simulink model "ModelRikiRollCalib"  (R2015b)
settings: Solver=ode45  StartTime=0.0  StopTime=3  MaxStep=Ts  RelTol=1e-3
model workspace (MAT data in the model file):
  MCOS : class17 (value not decoded)
  MCOS : class17 (value not decoded)
  MCOS : class17 (value not decoded)
  MCOS : class17 (value not decoded)
  MCOS : class17 (value not decoded)
values from neighbouring files (symbols this model uses):
  AltKp = 0.03    [params.mat]
  AltRateBias = 0.65    [params.mat]
  AltRateKi = 0.01    [params.mat]
  AltRateKp = 0.05    [params.mat]
  AltRateMax = 6    [params.mat]
  FilterK = [0.01 0.01 0.01 0.01 0.01 0.01 0.01 0.01 0.01 0.01 0.01 0.01 ... (100 elements, 1x100)]    [params.mat]
  PosKp = 0.1    [params.mat]
  RollPitchKp = 10    [params.mat]
  RollPitchMax = 30    [params.mat]
  RollPitchRateKd = 5e-05    [params.mat]
  RollPitchRateKi = 0.002    [params.mat]
  RollPitchRateKp = 0.0007    [params.mat]
  RollPitchRateMax = 200    [params.mat]
  VelKi = 0.02    [params.mat]
  VelKp = 0.15    [params.mat]
  VelMax = 6    [params.mat]
  Waypts = [10 20 50 50 50 50 200 20 20 0 0 50 ... (27 elements, 9x3)]    [params.mat]
  YawKp = 3    [params.mat]
  YawRateKi = 0.000213867089849    [params.mat]
  YawRateKp = 0.00321759853461    [params.mat]
  YawRateMax = 180    [params.mat]
undefined symbols (not defined in the file or in its folder): DiscIntNeverNeededParam, Earth, Receive, RollPitchKd, Send, sigbuilder_block, WGS84
libraries: simulink x49, aerolibutil x8, simulink_extras x6, aerolibfltsims x5, aerolibanimutils x2, aerolibtransform2 x2, aerolibconvert2 x2, aerolib6dof2 x1, aerolibatmos2 x1
(part 2 of 3)

== system ModelRikiRollCalib/Ctrl/AutoCtrl/Roll Controller ==
  BUS : Inport
  RollRef : Inport  Port=2
  Bus Selector1 : BusSelector  OutputSignals=RPY,dRPY
  Discrete PID Controller : simulink/Continuous/PID Controller  Controller=PI  TimeDomain=Discrete-time  SampleTime=Ts  IntegratorMethod=Forward Euler  FilterMethod=Forward Euler  Form=Parallel  UseFilter=on  ControllerParametersSource=internal  P=RollPitchRateKp  I=RollPitchRateKi  D=0  N=50  InitialConditionSource=internal  InitialConditionForIntegrator=0  InitialConditionForFilter=0  ExternalReset=none  LimitOutput=on  UpperSaturationLimit=0.2  LowerSaturationLimit=-0.2  LinearizeAsGain=off  AntiWindupMode=clamping  Kb=1  TrackingMode=off  Kt=1  PParamMin=[]  PParamMax=[]  IParamMin=[]  IParamMax=[]  DParamMin=[]  DParamMax=[]  NParamMin=[]  NParamMax=[]  KbParamMin=[]  KbParamMax=[]  KtParamMin=[]  KtParamMax=[]  POutMin=[]  POutMax=[]  IOutMin=[]  IOutMax=[]  DOutMin=[]  DOutMax=[]  NOutMin=[]  NOutMax=[]  KbOutMin=[]  KbOutMax=[]  KtOutMin=[]  KtOutMax=[]  IntegratorOutMin=[]  IntegratorOutMax=[]  FilterOutMin=[]  FilterOutMax=[]  SumOutMin=[]  SumOutMax=[]  SumI1OutMin=[]  SumI1OutMax=[]  SumI2OutMin=[]  SumI2OutMax=[]  SumI3OutMin=[]  SumI3OutMax=[]  SumDOutMin=[]  SumDOutMax=[]  SaturationOutMin=[]  SaturationOutMax=[]  IntegratorContinuousStateAttributes=''  IntegratorStateMustResolveToSignalObject=off  IntegratorRTWStateStorageClass=Auto  FilterContinuousStateAttributes=''  FilterStateMustResolveToSignalObject=off  FilterRTWStateStorageClass=Auto  DifferentiatorICPrevScaledInput=0  DifferentiatorOutMin=[]  DifferentiatorOutMax=[]
  Discrete PID Controller1 : simulink/Continuous/PID Controller  Controller=P  TimeDomain=Discrete-time  SampleTime=Ts  IntegratorMethod=Forward Euler  FilterMethod=Forward Euler  Form=Parallel  UseFilter=on  ControllerParametersSource=internal  P=RollPitchKp  I=0.0227534008426031  D=0  N=50  InitialConditionSource=internal  InitialConditionForIntegrator=0  InitialConditionForFilter=0  ExternalReset=none  LimitOutput=on  UpperSaturationLimit=RollPitchRateMax  LowerSaturationLimit=-RollPitchRateMax  LinearizeAsGain=off  AntiWindupMode=clamping  Kb=1  TrackingMode=off  Kt=1  PParamMin=[]  PParamMax=[]  IParamMin=[]  IParamMax=[]  DParamMin=[]  DParamMax=[]  NParamMin=[]  NParamMax=[]  KbParamMin=[]  KbParamMax=[]  KtParamMin=[]  KtParamMax=[]  POutMin=[]  POutMax=[]  IOutMin=[]  IOutMax=[]  DOutMin=[]  DOutMax=[]  NOutMin=[]  NOutMax=[]  KbOutMin=[]  KbOutMax=[]  KtOutMin=[]  KtOutMax=[]  IntegratorOutMin=[]  IntegratorOutMax=[]  FilterOutMin=[]  FilterOutMax=[]  SumOutMin=[]  SumOutMax=[]  SumI1OutMin=[]  SumI1OutMax=[]  SumI2OutMin=[]  SumI2OutMax=[]  SumI3OutMin=[]  SumI3OutMax=[]  SumDOutMin=[]  SumDOutMax=[]  SaturationOutMin=[]  SaturationOutMax=[]  IntegratorContinuousStateAttributes=''  IntegratorStateMustResolveToSignalObject=off  IntegratorRTWStateStorageClass=Auto  FilterContinuousStateAttributes=''  FilterStateMustResolveToSignalObject=off  FilterRTWStateStorageClass=Auto  DifferentiatorICPrevScaledInput=0  DifferentiatorOutMin=[]  DifferentiatorOutMax=[]
  Scale roll2 : Gain  Gain=RollPitchMax
  Selector : Selector  InputPortWidth=3  IndexOptions=Index vector (dialog)  Indices=[1]  OutputSizes=1
  Selector3 : Selector  InputPortWidth=3  IndexOptions=Index vector (dialog)  Indices=[1]  OutputSizes=1
  Sum : Sum  Inputs=|+-
  Sum3 : Sum  Inputs=|+-
  RollPWM : Outport
  wires:
  Scale roll2/1 -> Sum3/1
  Sum3/1 -> Discrete PID Controller1/1
  Selector3/1 -> Sum3/2
  Discrete PID Controller1/1 -> Sum/1
  Bus Selector1/1 -> Selector3/1  "<RPY>"
  Sum/1 -> Discrete PID Controller/1
  RollRef/1 -> Scale roll2/1
  Discrete PID Controller/1 -> RollPWM/1
  Selector/1 -> Sum/2  "dRoll"
  Bus Selector1/2 -> Selector/1  "<dRPY>"
  BUS/1 -> Bus Selector1/1

== system ModelRikiRollCalib/Ctrl/AutoCtrl/Subsystem ==
  AltRef : Inport
  VertVel : Inport  Port=2
  Altitude : Inport  Port=3
  Bias1 : Bias  Bias=AltRateBias
  Discrete PID Controller1 : simulink/Continuous/PID Controller  Controller=PI  TimeDomain=Discrete-time  SampleTime=Ts  IntegratorMethod=Forward Euler  FilterMethod=Forward Euler  Form=Parallel  UseFilter=on  ControllerParametersSource=internal  P=AltRateKp  I=AltRateKi  D=0  N=50  InitialConditionSource=internal  InitialConditionForIntegrator=0  InitialConditionForFilter=0  ExternalReset=none  LimitOutput=on  UpperSaturationLimit=0.5  LowerSaturationLimit=-0.5  LinearizeAsGain=off  AntiWindupMode=clamping  Kb=1  TrackingMode=off  Kt=1  PParamMin=[]  PParamMax=[]  IParamMin=[]  IParamMax=[]  DParamMin=[]  DParamMax=[]  NParamMin=[]  NParamMax=[]  KbParamMin=[]  KbParamMax=[]  KtParamMin=[]  KtParamMax=[]  POutMin=[]  POutMax=[]  IOutMin=[]  IOutMax=[]  DOutMin=[]  DOutMax=[]  NOutMin=[]  NOutMax=[]  KbOutMin=[]  KbOutMax=[]  KtOutMin=[]  KtOutMax=[]  IntegratorOutMin=[]  IntegratorOutMax=[]  FilterOutMin=[]  FilterOutMax=[]  SumOutMin=[]  SumOutMax=[]  SumI1OutMin=[]  SumI1OutMax=[]  SumI2OutMin=[]  SumI2OutMax=[]  SumI3OutMin=[]  SumI3OutMax=[]  SumDOutMin=[]  SumDOutMax=[]  SaturationOutMin=[]  SaturationOutMax=[]  IntegratorContinuousStateAttributes=''  IntegratorStateMustResolveToSignalObject=off  IntegratorRTWStateStorageClass=Auto  FilterContinuousStateAttributes=''  FilterStateMustResolveToSignalObject=off  FilterRTWStateStorageClass=Auto  DifferentiatorICPrevScaledInput=0  DifferentiatorOutMin=[]  DifferentiatorOutMax=[]
  Discrete PID Controller2 : simulink/Continuous/PID Controller  Controller=P  TimeDomain=Discrete-time  SampleTime=Ts  IntegratorMethod=Forward Euler  FilterMethod=Forward Euler  Form=Parallel  UseFilter=on  ControllerParametersSource=internal  P=AltKp  I=AltRateKi  D=0  N=50  InitialConditionSource=internal  InitialConditionForIntegrator=0  InitialConditionForFilter=0  ExternalReset=none  LimitOutput=on  UpperSaturationLimit=0.5  LowerSaturationLimit=-0.5  LinearizeAsGain=off  AntiWindupMode=clamping  Kb=1  TrackingMode=off  Kt=1  PParamMin=[]  PParamMax=[]  IParamMin=[]  IParamMax=[]  DParamMin=[]  DParamMax=[]  NParamMin=[]  NParamMax=[]  KbParamMin=[]  KbParamMax=[]  KtParamMin=[]  KtParamMax=[]  POutMin=[]  POutMax=[]  IOutMin=[]  IOutMax=[]  DOutMin=[]  DOutMax=[]  NOutMin=[]  NOutMax=[]  KbOutMin=[]  KbOutMax=[]  KtOutMin=[]  KtOutMax=[]  IntegratorOutMin=[]  IntegratorOutMax=[]  FilterOutMin=[]  FilterOutMax=[]  SumOutMin=[]  SumOutMax=[]  SumI1OutMin=[]  SumI1OutMax=[]  SumI2OutMin=[]  SumI2OutMax=[]  SumI3OutMin=[]  SumI3OutMax=[]  SumDOutMin=[]  SumDOutMax=[]  SaturationOutMin=[]  SaturationOutMax=[]  IntegratorContinuousStateAttributes=''  IntegratorStateMustResolveToSignalObject=off  IntegratorRTWStateStorageClass=Auto  FilterContinuousStateAttributes=''  FilterStateMustResolveToSignalObject=off  FilterRTWStateStorageClass=Auto  DifferentiatorICPrevScaledInput=0  DifferentiatorOutMin=[]  DifferentiatorOutMax=[]
  Scale Vel : Gain  Gain=AltRateMax*2
  Sum1 : Sum  Inputs=|+-
  Sum3 : Sum  Inputs=|+-
  Out1 : Outport
  wires:
  Bias1/1 -> Out1/1
  Scale Vel/1 -> Sum3/1
  VertVel/1 -> Sum3/2
  Discrete PID Controller1/1 -> Bias1/1
  Sum3/1 -> Discrete PID Controller1/1
  AltRef/1 -> Sum1/1
  Altitude/1 -> Sum1/2
  Discrete PID Controller2/1 -> Scale Vel/1
  Sum1/1 -> Discrete PID Controller2/1

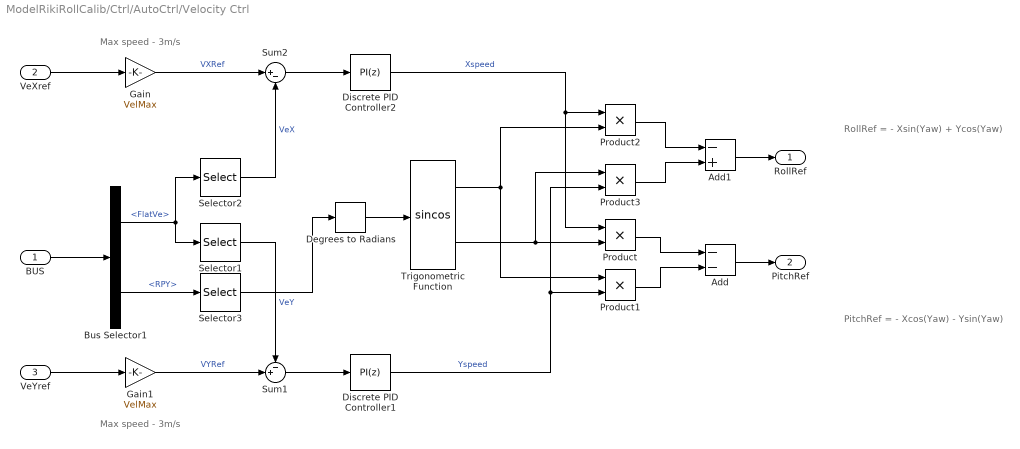
== system ModelRikiRollCalib/Ctrl/AutoCtrl/Velocity Ctrl ==
  note: Max speed - 3m/s
  note: PitchRef = - Xcos(Yaw) - Ysin(Yaw)
  note: RollRef = - Xsin(Yaw) + Ycos(Yaw)
  note: Max speed - 3m/s
  BUS : Inport
  VeXref : Inport  Port=2
  VeYref : Inport  Port=3
  Add : Sum  Inputs=--
  Add1 : Sum  Inputs=-+
  Bus Selector1 : BusSelector  OutputSignals=FlatVe,RPY
  Degrees to Radians : simulink_extras/Transformations/Degrees to Radians
  Discrete PID Controller1 : simulink/Continuous/PID Controller  Controller=PI  TimeDomain=Discrete-time  SampleTime=Ts  IntegratorMethod=Forward Euler  FilterMethod=Forward Euler  Form=Parallel  UseFilter=on  ControllerParametersSource=internal  P=VelKp  I=VelKi  D=0  N=50  InitialConditionSource=internal  InitialConditionForIntegrator=0  InitialConditionForFilter=0  ExternalReset=none  LimitOutput=on  UpperSaturationLimit=1  LowerSaturationLimit=-1  LinearizeAsGain=off  AntiWindupMode=clamping  Kb=1  TrackingMode=off  Kt=1  PParamMin=[]  PParamMax=[]  IParamMin=[]  IParamMax=[]  DParamMin=[]  DParamMax=[]  NParamMin=[]  NParamMax=[]  KbParamMin=[]  KbParamMax=[]  KtParamMin=[]  KtParamMax=[]  POutMin=[]  POutMax=[]  IOutMin=[]  IOutMax=[]  DOutMin=[]  DOutMax=[]  NOutMin=[]  NOutMax=[]  KbOutMin=[]  KbOutMax=[]  KtOutMin=[]  KtOutMax=[]  IntegratorOutMin=[]  IntegratorOutMax=[]  FilterOutMin=[]  FilterOutMax=[]  SumOutMin=[]  SumOutMax=[]  SumI1OutMin=[]  SumI1OutMax=[]  SumI2OutMin=[]  SumI2OutMax=[]  SumI3OutMin=[]  SumI3OutMax=[]  SumDOutMin=[]  SumDOutMax=[]  SaturationOutMin=[]  SaturationOutMax=[]  IntegratorContinuousStateAttributes=''  IntegratorStateMustResolveToSignalObject=off  IntegratorRTWStateStorageClass=Auto  FilterContinuousStateAttributes=''  FilterStateMustResolveToSignalObject=off  FilterRTWStateStorageClass=Auto  DifferentiatorICPrevScaledInput=0  DifferentiatorOutMin=[]  DifferentiatorOutMax=[]
  Discrete PID Controller2 : simulink/Continuous/PID Controller  Controller=PI  TimeDomain=Discrete-time  SampleTime=Ts  IntegratorMethod=Forward Euler  FilterMethod=Forward Euler  Form=Parallel  UseFilter=on  ControllerParametersSource=internal  P=VelKp  I=VelKi  D=0  N=50  InitialConditionSource=internal  InitialConditionForIntegrator=0  InitialConditionForFilter=0  ExternalReset=none  LimitOutput=on  UpperSaturationLimit=1  LowerSaturationLimit=-1  LinearizeAsGain=off  AntiWindupMode=clamping  Kb=1  TrackingMode=off  Kt=1  PParamMin=[]  PParamMax=[]  IParamMin=[]  IParamMax=[]  DParamMin=[]  DParamMax=[]  NParamMin=[]  NParamMax=[]  KbParamMin=[]  KbParamMax=[]  KtParamMin=[]  KtParamMax=[]  POutMin=[]  POutMax=[]  IOutMin=[]  IOutMax=[]  DOutMin=[]  DOutMax=[]  NOutMin=[]  NOutMax=[]  KbOutMin=[]  KbOutMax=[]  KtOutMin=[]  KtOutMax=[]  IntegratorOutMin=[]  IntegratorOutMax=[]  FilterOutMin=[]  FilterOutMax=[]  SumOutMin=[]  SumOutMax=[]  SumI1OutMin=[]  SumI1OutMax=[]  SumI2OutMin=[]  SumI2OutMax=[]  SumI3OutMin=[]  SumI3OutMax=[]  SumDOutMin=[]  SumDOutMax=[]  SaturationOutMin=[]  SaturationOutMax=[]  IntegratorContinuousStateAttributes=''  IntegratorStateMustResolveToSignalObject=off  IntegratorRTWStateStorageClass=Auto  FilterContinuousStateAttributes=''  FilterStateMustResolveToSignalObject=off  FilterRTWStateStorageClass=Auto  DifferentiatorICPrevScaledInput=0  DifferentiatorOutMin=[]  DifferentiatorOutMax=[]
  Gain : Gain  Gain=VelMax
  Gain1 : Gain  Gain=VelMax
  Product{,1..3} (4 alike) : Product  RndMeth=Zero
  Selector1 : Selector  InputPortWidth=3  IndexOptions=Index vector (dialog)  Indices=[2]  OutputSizes=1
  Selector2 : Selector  InputPortWidth=3  IndexOptions=Index vector (dialog)  Indices=[1]  OutputSizes=1
  Selector3 : Selector  InputPortWidth=3  IndexOptions=Index vector (dialog)  Indices=[3]  OutputSizes=1
  Sum1 : Sum  Inputs=-+|
  Sum2 : Sum  Inputs=|+-
  Trigonometric Function : Trigonometry  Operator=sincos
  RollRef : Outport
  PitchRef : Outport  Port=2
  wires:
  VeXref/1 -> Gain/1
  Selector2/1 -> Sum2/2  "VeX"
  Sum2/1 -> Discrete PID Controller2/1
  Bus Selector1/1 -> Selector1/1, Selector2/1  "<FlatVe>"
  BUS/1 -> Bus Selector1/1
  VeYref/1 -> Gain1/1
  Selector1/1 -> Sum1/1  "VeY"
  Sum1/1 -> Discrete PID Controller1/1
  Discrete PID Controller2/1 -> Product/1, Product2/1  "Xspeed"
  Discrete PID Controller1/1 -> Product1/2, Product3/2  "Yspeed"
  Trigonometric Function/2 -> Product/2, Product3/1
  Trigonometric Function/1 -> Product1/1, Product2/2
  Product1/1 -> Add/2
  Product/1 -> Add/1
  Product2/1 -> Add1/1
  Product3/1 -> Add1/2
  Add1/1 -> RollRef/1
  Add/1 -> PitchRef/1
  Bus Selector1/2 -> Selector3/1  "<RPY>"
  Selector3/1 -> Degrees to Radians/1
  Gain/1 -> Sum2/1  "VXRef"
  Gain1/1 -> Sum1/2  "VYRef"
  Degrees to Radians/1 -> Trigonometric Function/1

== system ModelRikiRollCalib/Ctrl/AutoCtrl/Yaw Controller ==
  BUS : Inport
  YawRef : Inport  Port=2
  Bus Selector3 : BusSelector  OutputSignals=RPY,dRPY
  Correct Yaw1 : MATLAB Function  TreatAsAtomicUnit=on
  Discrete PID Controller : simulink/Continuous/PID Controller  Controller=PI  TimeDomain=Discrete-time  SampleTime=Ts  IntegratorMethod=Forward Euler  FilterMethod=Forward Euler  Form=Parallel  UseFilter=on  ControllerParametersSource=internal  P=YawRateKp  I=YawRateKi  D=0  N=10  InitialConditionSource=internal  InitialConditionForIntegrator=0  InitialConditionForFilter=0  ExternalReset=none  LimitOutput=on  UpperSaturationLimit=0.2  LowerSaturationLimit=-0.2  LinearizeAsGain=off  AntiWindupMode=clamping  Kb=1  TrackingMode=off  Kt=1  PParamMin=[]  PParamMax=[]  IParamMin=[]  IParamMax=[]  DParamMin=[]  DParamMax=[]  NParamMin=[]  NParamMax=[]  KbParamMin=[]  KbParamMax=[]  KtParamMin=[]  KtParamMax=[]  POutMin=[]  POutMax=[]  IOutMin=[]  IOutMax=[]  DOutMin=[]  DOutMax=[]  NOutMin=[]  NOutMax=[]  KbOutMin=[]  KbOutMax=[]  KtOutMin=[]  KtOutMax=[]  IntegratorOutMin=[]  IntegratorOutMax=[]  FilterOutMin=[]  FilterOutMax=[]  SumOutMin=[]  SumOutMax=[]  SumI1OutMin=[]  SumI1OutMax=[]  SumI2OutMin=[]  SumI2OutMax=[]  SumI3OutMin=[]  SumI3OutMax=[]  SumDOutMin=[]  SumDOutMax=[]  SaturationOutMin=[]  SaturationOutMax=[]  IntegratorContinuousStateAttributes=''  IntegratorStateMustResolveToSignalObject=off  IntegratorRTWStateStorageClass=Auto  FilterContinuousStateAttributes=''  FilterStateMustResolveToSignalObject=off  FilterRTWStateStorageClass=Auto  DifferentiatorICPrevScaledInput=0  DifferentiatorOutMin=[]  DifferentiatorOutMax=[]
  Discrete PID Controller3 : simulink/Continuous/PID Controller  Controller=P  TimeDomain=Discrete-time  SampleTime=Ts  IntegratorMethod=Forward Euler  FilterMethod=Forward Euler  Form=Parallel  UseFilter=on  ControllerParametersSource=internal  P=YawKp  I=0  D=0  N=10  InitialConditionSource=internal  InitialConditionForIntegrator=0  InitialConditionForFilter=0  ExternalReset=none  LimitOutput=on  UpperSaturationLimit=YawRateMax  LowerSaturationLimit=-YawRateMax  LinearizeAsGain=off  AntiWindupMode=clamping  Kb=1  TrackingMode=off  Kt=1  PParamMin=[]  PParamMax=[]  IParamMin=[]  IParamMax=[]  DParamMin=[]  DParamMax=[]  NParamMin=[]  NParamMax=[]  KbParamMin=[]  KbParamMax=[]  KtParamMin=[]  KtParamMax=[]  POutMin=[]  POutMax=[]  IOutMin=[]  IOutMax=[]  DOutMin=[]  DOutMax=[]  NOutMin=[]  NOutMax=[]  KbOutMin=[]  KbOutMax=[]  KtOutMin=[]  KtOutMax=[]  IntegratorOutMin=[]  IntegratorOutMax=[]  FilterOutMin=[]  FilterOutMax=[]  SumOutMin=[]  SumOutMax=[]  SumI1OutMin=[]  SumI1OutMax=[]  SumI2OutMin=[]  SumI2OutMax=[]  SumI3OutMin=[]  SumI3OutMax=[]  SumDOutMin=[]  SumDOutMax=[]  SaturationOutMin=[]  SaturationOutMax=[]  IntegratorContinuousStateAttributes=''  IntegratorStateMustResolveToSignalObject=off  IntegratorRTWStateStorageClass=Auto  FilterContinuousStateAttributes=''  FilterStateMustResolveToSignalObject=off  FilterRTWStateStorageClass=Auto  DifferentiatorICPrevScaledInput=0  DifferentiatorOutMin=[]  DifferentiatorOutMax=[]
  Discrete-Time Integrator : DiscreteIntegrator  SampleTime=Ts  ICPrevOutput=DiscIntNeverNeededParam  ICPrevScaledInput=DiscIntNeverNeededParam
  Scale roll2 : Gain  Gain=90
  Selector : Selector  InputPortWidth=3  IndexOptions=Index vector (dialog)  Indices=[3]  OutputSizes=1
  Selector2 : Selector  InputPortWidth=3  IndexOptions=Index vector (dialog)  Indices=[3]  OutputSizes=1
  Sum : Sum  Inputs=|+-
  Sum3 : Sum  Inputs=|+-
  YawPWM : Outport
  wires:
  Scale roll2/1 -> Discrete-Time Integrator/1
  Selector2/1 -> Sum3/2
  YawRef/1 -> Scale roll2/1
  Bus Selector3/1 -> Selector2/1  "<RPY>"
  BUS/1 -> Bus Selector3/1
  Bus Selector3/2 -> Selector/1  "<dRPY>"
  Correct Yaw1/1(y) -> Discrete PID Controller3/1
  Discrete PID Controller3/1 -> Sum/1
  Sum3/1 -> Correct Yaw1/1(u)
  Selector/1 -> Sum/2  "dYaw"
  Sum/1 -> Discrete PID Controller/1
  Discrete PID Controller/1 -> YawPWM/1
  Discrete-Time Integrator/1 -> Sum3/1

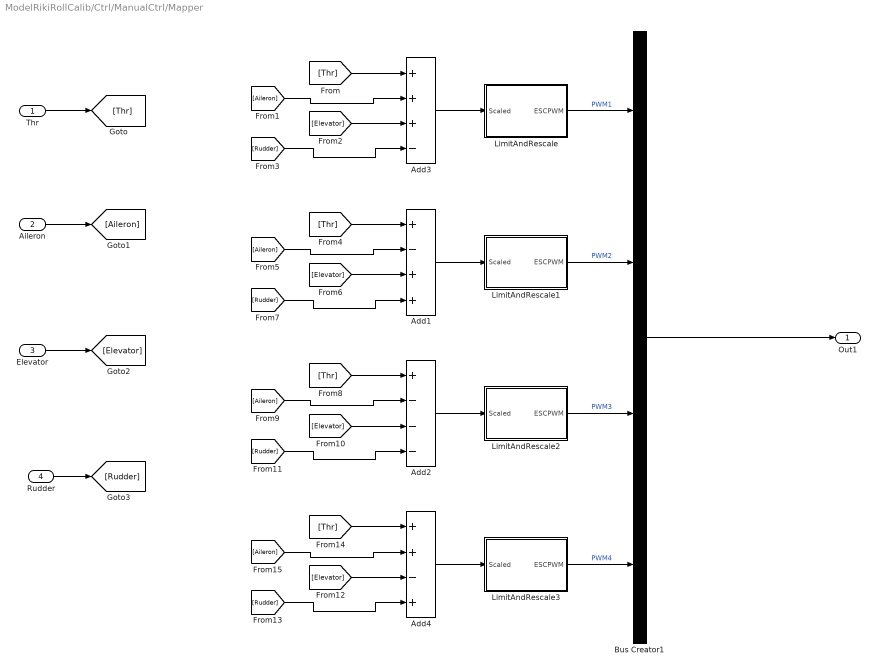
== system ModelRikiRollCalib/Ctrl/ManualCtrl/Mapper ==
  Thr : Inport
  Aileron : Inport  Port=2
  Elevator : Inport  Port=3
  Rudder : Inport  Port=4
  Add1 : Sum  Inputs=+-++
  Add2 : Sum  Inputs=+---
  Add3 : Sum  Inputs=+++-
  Add4 : Sum  Inputs=++-+
  Bus Creator1 : BusCreator  Inputs=4
  LimitAndRescale : Subsystem
  LimitAndRescale1 : Subsystem
  LimitAndRescale2 : Subsystem
  LimitAndRescale3 : Subsystem
  Out1 : Outport
  wires:
  LimitAndRescale3/1(ESCPWM) -> Bus Creator1/4  "PWM4"
  Add4/1 -> LimitAndRescale3/1(Scaled)
  LimitAndRescale2/1(ESCPWM) -> Bus Creator1/3  "PWM3"
  Add2/1 -> LimitAndRescale2/1(Scaled)
  Bus Creator1/1 -> Out1/1
  LimitAndRescale/1(ESCPWM) -> Bus Creator1/1  "PWM1"
  Add3/1 -> LimitAndRescale/1(Scaled)
  LimitAndRescale1/1(ESCPWM) -> Bus Creator1/2  "PWM2"
  Thr/1 -> [Thr]
  Aileron/1 -> [Aileron]
  Elevator/1 -> [Elevator]
  Rudder/1 -> [Rudder]
  [Thr] -> Add3/1
  [Aileron] -> Add3/2
  [Elevator] -> Add3/3
  [Rudder] -> Add3/4
  Add1/1 -> LimitAndRescale1/1(Scaled)
  [Thr] -> Add1/1
  [Aileron] -> Add1/2
  [Elevator] -> Add1/3
  [Rudder] -> Add1/4
  [Thr] -> Add2/1
  [Aileron] -> Add2/2
  [Elevator] -> Add2/3
  [Rudder] -> Add2/4
  [Thr] -> Add4/1
  [Aileron] -> Add4/2
  [Elevator] -> Add4/3
  [Rudder] -> Add4/4

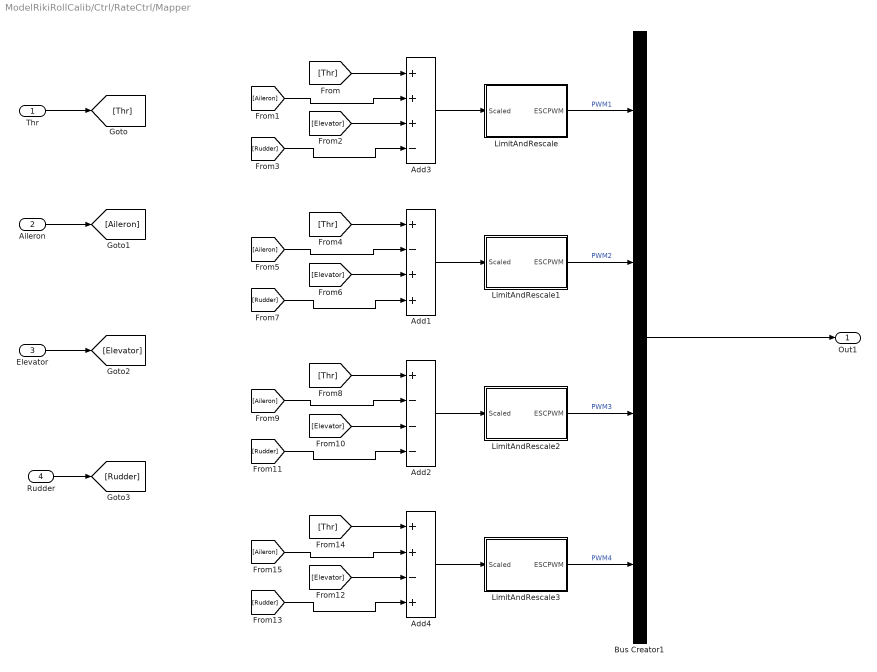
== system ModelRikiRollCalib/Ctrl/RateCtrl/Mapper ==
  Thr : Inport
  Aileron : Inport  Port=2
  Elevator : Inport  Port=3
  Rudder : Inport  Port=4
  Add1 : Sum  Inputs=+-++
  Add2 : Sum  Inputs=+---
  Add3 : Sum  Inputs=+++-
  Add4 : Sum  Inputs=++-+
  Bus Creator1 : BusCreator  Inputs=4
  LimitAndRescale : Subsystem
  LimitAndRescale1 : Subsystem
  LimitAndRescale2 : Subsystem
  LimitAndRescale3 : Subsystem
  Out1 : Outport
  wires:
  LimitAndRescale3/1(ESCPWM) -> Bus Creator1/4  "PWM4"
  Add4/1 -> LimitAndRescale3/1(Scaled)
  LimitAndRescale2/1(ESCPWM) -> Bus Creator1/3  "PWM3"
  Add2/1 -> LimitAndRescale2/1(Scaled)
  Bus Creator1/1 -> Out1/1
  LimitAndRescale/1(ESCPWM) -> Bus Creator1/1  "PWM1"
  Add3/1 -> LimitAndRescale/1(Scaled)
  LimitAndRescale1/1(ESCPWM) -> Bus Creator1/2  "PWM2"
  Thr/1 -> [Thr]
  Aileron/1 -> [Aileron]
  Elevator/1 -> [Elevator]
  Rudder/1 -> [Rudder]
  [Thr] -> Add3/1
  [Aileron] -> Add3/2
  [Elevator] -> Add3/3
  [Rudder] -> Add3/4
  Add1/1 -> LimitAndRescale1/1(Scaled)
  [Thr] -> Add1/1
  [Aileron] -> Add1/2
  [Elevator] -> Add1/3
  [Rudder] -> Add1/4
  [Thr] -> Add2/1
  [Aileron] -> Add2/2
  [Elevator] -> Add2/3
  [Rudder] -> Add2/4
  [Thr] -> Add4/1
  [Aileron] -> Add4/2
  [Elevator] -> Add4/3
  [Rudder] -> Add4/4

== system ModelRikiRollCalib/Ctrl/RateCtrl/Pitch Controller ==
  BUS : Inport
  PitchRef : Inport  Port=2
  Bus Selector1 : BusSelector  OutputSignals=dRPY
  Discrete PID Controller : simulink/Continuous/PID Controller  Controller=PI  TimeDomain=Discrete-time  SampleTime=Ts  IntegratorMethod=Forward Euler  FilterMethod=Forward Euler  Form=Parallel  UseFilter=on  ControllerParametersSource=internal  P=RollPitchRateKp  I=RollPitchRateKi  D=0  N=50  InitialConditionSource=internal  InitialConditionForIntegrator=0  InitialConditionForFilter=0  ExternalReset=none  LimitOutput=on  UpperSaturationLimit=0.2  LowerSaturationLimit=-0.2  LinearizeAsGain=off  AntiWindupMode=clamping  Kb=1  TrackingMode=off  Kt=1  PParamMin=[]  PParamMax=[]  IParamMin=[]  IParamMax=[]  DParamMin=[]  DParamMax=[]  NParamMin=[]  NParamMax=[]  KbParamMin=[]  KbParamMax=[]  KtParamMin=[]  KtParamMax=[]  POutMin=[]  POutMax=[]  IOutMin=[]  IOutMax=[]  DOutMin=[]  DOutMax=[]  NOutMin=[]  NOutMax=[]  KbOutMin=[]  KbOutMax=[]  KtOutMin=[]  KtOutMax=[]  IntegratorOutMin=[]  IntegratorOutMax=[]  FilterOutMin=[]  FilterOutMax=[]  SumOutMin=[]  SumOutMax=[]  SumI1OutMin=[]  SumI1OutMax=[]  SumI2OutMin=[]  SumI2OutMax=[]  SumI3OutMin=[]  SumI3OutMax=[]  SumDOutMin=[]  SumDOutMax=[]  SaturationOutMin=[]  SaturationOutMax=[]  IntegratorContinuousStateAttributes=''  IntegratorStateMustResolveToSignalObject=off  IntegratorRTWStateStorageClass=Auto  FilterContinuousStateAttributes=''  FilterStateMustResolveToSignalObject=off  FilterRTWStateStorageClass=Auto  DifferentiatorICPrevScaledInput=0  DifferentiatorOutMin=[]  DifferentiatorOutMax=[]
  Scale roll2 : Gain  Gain=RollPitchRateMax
  Selector : Selector  InputPortWidth=3  IndexOptions=Index vector (dialog)  Indices=[2]  OutputSizes=1
  Sum : Sum  Inputs=|+-
  PitchPWM : Outport
  wires:
  Scale roll2/1 -> Sum/1
  Sum/1 -> Discrete PID Controller/1
  PitchRef/1 -> Scale roll2/1
  Discrete PID Controller/1 -> PitchPWM/1
  Selector/1 -> Sum/2  "dPitch"
  Bus Selector1/1 -> Selector/1  "<dRPY>"
  BUS/1 -> Bus Selector1/1

== system ModelRikiRollCalib/Ctrl/RateCtrl/Roll Controller ==
  BUS : Inport
  RollRef : Inport  Port=2
  Bus Selector1 : BusSelector  OutputSignals=dRPY
  Discrete PID Controller : simulink/Continuous/PID Controller  Controller=PD  TimeDomain=Discrete-time  SampleTime=Ts  IntegratorMethod=Forward Euler  FilterMethod=Forward Euler  Form=Parallel  UseFilter=on  ControllerParametersSource=internal  P=RollPitchRateKp  I=RollPitchRateKi  D=RollPitchRateKd  N=50  InitialConditionSource=internal  InitialConditionForIntegrator=0  InitialConditionForFilter=0  ExternalReset=none  LimitOutput=on  UpperSaturationLimit=0.2  LowerSaturationLimit=-0.2  LinearizeAsGain=off  AntiWindupMode=clamping  Kb=1  TrackingMode=off  Kt=1  PParamMin=[]  PParamMax=[]  IParamMin=[]  IParamMax=[]  DParamMin=[]  DParamMax=[]  NParamMin=[]  NParamMax=[]  KbParamMin=[]  KbParamMax=[]  KtParamMin=[]  KtParamMax=[]  POutMin=[]  POutMax=[]  IOutMin=[]  IOutMax=[]  DOutMin=[]  DOutMax=[]  NOutMin=[]  NOutMax=[]  KbOutMin=[]  KbOutMax=[]  KtOutMin=[]  KtOutMax=[]  IntegratorOutMin=[]  IntegratorOutMax=[]  FilterOutMin=[]  FilterOutMax=[]  SumOutMin=[]  SumOutMax=[]  SumI1OutMin=[]  SumI1OutMax=[]  SumI2OutMin=[]  SumI2OutMax=[]  SumI3OutMin=[]  SumI3OutMax=[]  SumDOutMin=[]  SumDOutMax=[]  SaturationOutMin=[]  SaturationOutMax=[]  IntegratorContinuousStateAttributes=''  IntegratorStateMustResolveToSignalObject=off  IntegratorRTWStateStorageClass=Auto  FilterContinuousStateAttributes=''  FilterStateMustResolveToSignalObject=off  FilterRTWStateStorageClass=Auto  DifferentiatorICPrevScaledInput=0  DifferentiatorOutMin=[]  DifferentiatorOutMax=[]
  Scale roll2 : Gain  Gain=RollPitchRateMax
  Selector : Selector  InputPortWidth=3  IndexOptions=Index vector (dialog)  Indices=[1]  OutputSizes=1
  Sum : Sum  Inputs=|+-
  RollPWM : Outport
  wires:
  BUS/1 -> Bus Selector1/1
  Bus Selector1/1 -> Selector/1  "<dRPY>"
  Selector/1 -> Sum/2  "dRoll"
  Discrete PID Controller/1 -> RollPWM/1  "RateRollY"
  RollRef/1 -> Scale roll2/1
  Sum/1 -> Discrete PID Controller/1
  Scale roll2/1 -> Sum/1  "RateRollRef"

== system ModelRikiRollCalib/Ctrl/RateCtrl/Yaw Controller ==
  BUS : Inport
  YawRef : Inport  Port=2
  Bus Selector1 : BusSelector  OutputSignals=dRPY
  Discrete PID Controller : simulink/Continuous/PID Controller  Controller=PI  TimeDomain=Discrete-time  SampleTime=Ts  IntegratorMethod=Forward Euler  FilterMethod=Forward Euler  Form=Parallel  UseFilter=on  ControllerParametersSource=internal  P=YawRateKp  I=YawRateKi  D=0  N=10  InitialConditionSource=internal  InitialConditionForIntegrator=0  InitialConditionForFilter=0  ExternalReset=none  LimitOutput=on  UpperSaturationLimit=0.2  LowerSaturationLimit=-0.2  LinearizeAsGain=off  AntiWindupMode=clamping  Kb=1  TrackingMode=off  Kt=1  PParamMin=[]  PParamMax=[]  IParamMin=[]  IParamMax=[]  DParamMin=[]  DParamMax=[]  NParamMin=[]  NParamMax=[]  KbParamMin=[]  KbParamMax=[]  KtParamMin=[]  KtParamMax=[]  POutMin=[]  POutMax=[]  IOutMin=[]  IOutMax=[]  DOutMin=[]  DOutMax=[]  NOutMin=[]  NOutMax=[]  KbOutMin=[]  KbOutMax=[]  KtOutMin=[]  KtOutMax=[]  IntegratorOutMin=[]  IntegratorOutMax=[]  FilterOutMin=[]  FilterOutMax=[]  SumOutMin=[]  SumOutMax=[]  SumI1OutMin=[]  SumI1OutMax=[]  SumI2OutMin=[]  SumI2OutMax=[]  SumI3OutMin=[]  SumI3OutMax=[]  SumDOutMin=[]  SumDOutMax=[]  SaturationOutMin=[]  SaturationOutMax=[]  IntegratorContinuousStateAttributes=''  IntegratorStateMustResolveToSignalObject=off  IntegratorRTWStateStorageClass=Auto  FilterContinuousStateAttributes=''  FilterStateMustResolveToSignalObject=off  FilterRTWStateStorageClass=Auto  DifferentiatorICPrevScaledInput=0  DifferentiatorOutMin=[]  DifferentiatorOutMax=[]
  Scale roll2 : Gain  Gain=YawRateMax
  Selector : Selector  InputPortWidth=3  IndexOptions=Index vector (dialog)  Indices=[3]  OutputSizes=1
  Sum : Sum  Inputs=|+-
  YawPWM : Outport
  wires:
  Scale roll2/1 -> Sum/1
  Sum/1 -> Discrete PID Controller/1
  YawRef/1 -> Scale roll2/1
  Discrete PID Controller/1 -> YawPWM/1
  Selector/1 -> Sum/2  "dYaw"
  Bus Selector1/1 -> Selector/1  "<dRPY>"
  BUS/1 -> Bus Selector1/1

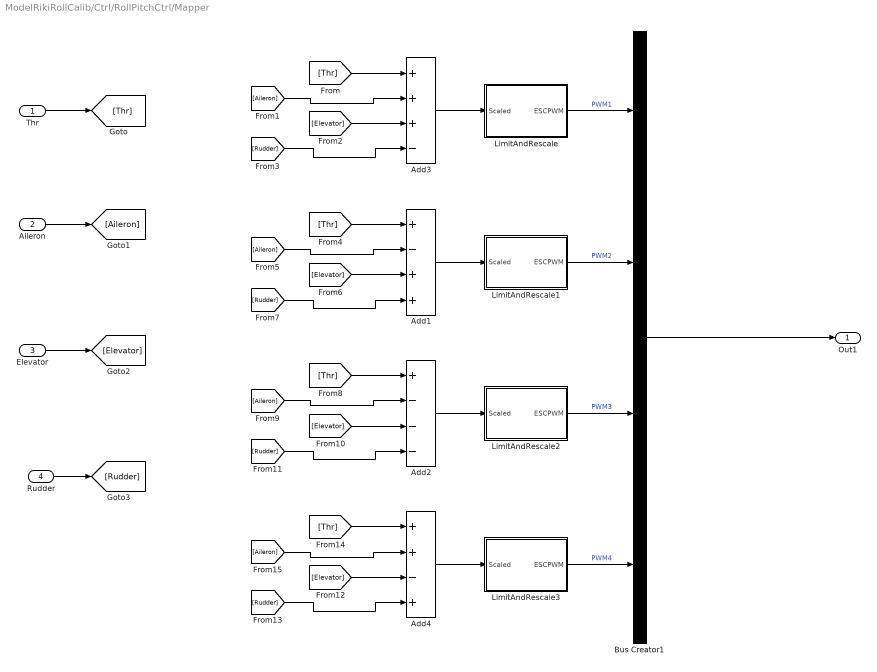
== system ModelRikiRollCalib/Ctrl/RollPitchCtrl/Mapper ==
  Thr : Inport
  Aileron : Inport  Port=2
  Elevator : Inport  Port=3
  Rudder : Inport  Port=4
  Add1 : Sum  Inputs=+-++
  Add2 : Sum  Inputs=+---
  Add3 : Sum  Inputs=+++-
  Add4 : Sum  Inputs=++-+
  Bus Creator1 : BusCreator  Inputs=4
  LimitAndRescale : Subsystem
  LimitAndRescale1 : Subsystem
  LimitAndRescale2 : Subsystem
  LimitAndRescale3 : Subsystem
  Out1 : Outport
  wires:
  LimitAndRescale3/1(ESCPWM) -> Bus Creator1/4  "PWM4"
  Add4/1 -> LimitAndRescale3/1(Scaled)
  LimitAndRescale2/1(ESCPWM) -> Bus Creator1/3  "PWM3"
  Add2/1 -> LimitAndRescale2/1(Scaled)
  Bus Creator1/1 -> Out1/1
  LimitAndRescale/1(ESCPWM) -> Bus Creator1/1  "PWM1"
  Add3/1 -> LimitAndRescale/1(Scaled)
  LimitAndRescale1/1(ESCPWM) -> Bus Creator1/2  "PWM2"
  Thr/1 -> [Thr]
  Aileron/1 -> [Aileron]
  Elevator/1 -> [Elevator]
  Rudder/1 -> [Rudder]
  [Thr] -> Add3/1
  [Aileron] -> Add3/2
  [Elevator] -> Add3/3
  [Rudder] -> Add3/4
  Add1/1 -> LimitAndRescale1/1(Scaled)
  [Thr] -> Add1/1
  [Aileron] -> Add1/2
  [Elevator] -> Add1/3
  [Rudder] -> Add1/4
  [Thr] -> Add2/1
  [Aileron] -> Add2/2
  [Elevator] -> Add2/3
  [Rudder] -> Add2/4
  [Thr] -> Add4/1
  [Aileron] -> Add4/2
  [Elevator] -> Add4/3
  [Rudder] -> Add4/4

== system ModelRikiRollCalib/Ctrl/RollPitchCtrl/Pitch Controller ==
  BUS : Inport
  PitchRef : Inport  Port=2
  Bus Selector2 : BusSelector  OutputSignals=RPY,dRPY
  Discrete PID Controller : simulink/Continuous/PID Controller  Controller=PI  TimeDomain=Discrete-time  SampleTime=Ts  IntegratorMethod=Forward Euler  FilterMethod=Forward Euler  Form=Parallel  UseFilter=on  ControllerParametersSource=internal  P=RollPitchRateKp  I=RollPitchRateKi  D=0  N=50  InitialConditionSource=internal  InitialConditionForIntegrator=0  InitialConditionForFilter=0  ExternalReset=none  LimitOutput=on  UpperSaturationLimit=0.2  LowerSaturationLimit=-0.2  LinearizeAsGain=off  AntiWindupMode=clamping  Kb=1  TrackingMode=off  Kt=1  PParamMin=[]  PParamMax=[]  IParamMin=[]  IParamMax=[]  DParamMin=[]  DParamMax=[]  NParamMin=[]  NParamMax=[]  KbParamMin=[]  KbParamMax=[]  KtParamMin=[]  KtParamMax=[]  POutMin=[]  POutMax=[]  IOutMin=[]  IOutMax=[]  DOutMin=[]  DOutMax=[]  NOutMin=[]  NOutMax=[]  KbOutMin=[]  KbOutMax=[]  KtOutMin=[]  KtOutMax=[]  IntegratorOutMin=[]  IntegratorOutMax=[]  FilterOutMin=[]  FilterOutMax=[]  SumOutMin=[]  SumOutMax=[]  SumI1OutMin=[]  SumI1OutMax=[]  SumI2OutMin=[]  SumI2OutMax=[]  SumI3OutMin=[]  SumI3OutMax=[]  SumDOutMin=[]  SumDOutMax=[]  SaturationOutMin=[]  SaturationOutMax=[]  IntegratorContinuousStateAttributes=''  IntegratorStateMustResolveToSignalObject=off  IntegratorRTWStateStorageClass=Auto  FilterContinuousStateAttributes=''  FilterStateMustResolveToSignalObject=off  FilterRTWStateStorageClass=Auto  DifferentiatorICPrevScaledInput=0  DifferentiatorOutMin=[]  DifferentiatorOutMax=[]
  Discrete PID Controller1 : simulink/Continuous/PID Controller  Controller=P  TimeDomain=Discrete-time  SampleTime=Ts  IntegratorMethod=Forward Euler  FilterMethod=Forward Euler  Form=Parallel  UseFilter=on  ControllerParametersSource=internal  P=RollPitchKp  I=0.0227534008426031  D=0  N=50  InitialConditionSource=internal  InitialConditionForIntegrator=0  InitialConditionForFilter=0  ExternalReset=none  LimitOutput=on  UpperSaturationLimit=RollPitchRateMax  LowerSaturationLimit=-RollPitchRateMax  LinearizeAsGain=off  AntiWindupMode=clamping  Kb=1  TrackingMode=off  Kt=1  PParamMin=[]  PParamMax=[]  IParamMin=[]  IParamMax=[]  DParamMin=[]  DParamMax=[]  NParamMin=[]  NParamMax=[]  KbParamMin=[]  KbParamMax=[]  KtParamMin=[]  KtParamMax=[]  POutMin=[]  POutMax=[]  IOutMin=[]  IOutMax=[]  DOutMin=[]  DOutMax=[]  NOutMin=[]  NOutMax=[]  KbOutMin=[]  KbOutMax=[]  KtOutMin=[]  KtOutMax=[]  IntegratorOutMin=[]  IntegratorOutMax=[]  FilterOutMin=[]  FilterOutMax=[]  SumOutMin=[]  SumOutMax=[]  SumI1OutMin=[]  SumI1OutMax=[]  SumI2OutMin=[]  SumI2OutMax=[]  SumI3OutMin=[]  SumI3OutMax=[]  SumDOutMin=[]  SumDOutMax=[]  SaturationOutMin=[]  SaturationOutMax=[]  IntegratorContinuousStateAttributes=''  IntegratorStateMustResolveToSignalObject=off  IntegratorRTWStateStorageClass=Auto  FilterContinuousStateAttributes=''  FilterStateMustResolveToSignalObject=off  FilterRTWStateStorageClass=Auto  DifferentiatorICPrevScaledInput=0  DifferentiatorOutMin=[]  DifferentiatorOutMax=[]
  Scale roll1 : Gain  Gain=RollPitchMax
  Selector1 : Selector  InputPortWidth=3  IndexOptions=Index vector (dialog)  Indices=[2]  OutputSizes=1
  Selector2 : Selector  InputPortWidth=3  IndexOptions=Index vector (dialog)  Indices=[2]  OutputSizes=1
  Sum1 : Sum  Inputs=|+-
  Sum3 : Sum  Inputs=|+-
  PitchPWM : Outport
  wires:
  BUS/1 -> Bus Selector2/1
  Bus Selector2/2 -> Selector2/1  "<dRPY>"
  Selector2/1 -> Sum1/2  "dRoll"
  Discrete PID Controller/1 -> PitchPWM/1
  PitchRef/1 -> Scale roll1/1
  Sum1/1 -> Discrete PID Controller/1
  Bus Selector2/1 -> Selector1/1  "<RPY>"
  Discrete PID Controller1/1 -> Sum1/1
  Selector1/1 -> Sum3/2
  Sum3/1 -> Discrete PID Controller1/1
  Scale roll1/1 -> Sum3/1

== system ModelRikiRollCalib/Ctrl/RollPitchCtrl/Roll Controller ==
  BUS : Inport
  RollRef : Inport  Port=2
  Bus Selector1 : BusSelector  OutputSignals=RPY,dRPY
  Discrete PID Controller : simulink/Continuous/PID Controller  Controller=PD  TimeDomain=Discrete-time  SampleTime=Ts  IntegratorMethod=Forward Euler  FilterMethod=Forward Euler  Form=Parallel  UseFilter=on  ControllerParametersSource=internal  P=RollPitchRateKp  I=RollPitchRateKi  D=RollPitchRateKd  N=50  InitialConditionSource=internal  InitialConditionForIntegrator=0  InitialConditionForFilter=0  ExternalReset=none  LimitOutput=on  UpperSaturationLimit=0.2  LowerSaturationLimit=-0.2  LinearizeAsGain=off  AntiWindupMode=clamping  Kb=1  TrackingMode=off  Kt=1  PParamMin=[]  PParamMax=[]  IParamMin=[]  IParamMax=[]  DParamMin=[]  DParamMax=[]  NParamMin=[]  NParamMax=[]  KbParamMin=[]  KbParamMax=[]  KtParamMin=[]  KtParamMax=[]  POutMin=[]  POutMax=[]  IOutMin=[]  IOutMax=[]  DOutMin=[]  DOutMax=[]  NOutMin=[]  NOutMax=[]  KbOutMin=[]  KbOutMax=[]  KtOutMin=[]  KtOutMax=[]  IntegratorOutMin=[]  IntegratorOutMax=[]  FilterOutMin=[]  FilterOutMax=[]  SumOutMin=[]  SumOutMax=[]  SumI1OutMin=[]  SumI1OutMax=[]  SumI2OutMin=[]  SumI2OutMax=[]  SumI3OutMin=[]  SumI3OutMax=[]  SumDOutMin=[]  SumDOutMax=[]  SaturationOutMin=[]  SaturationOutMax=[]  IntegratorContinuousStateAttributes=''  IntegratorStateMustResolveToSignalObject=off  IntegratorRTWStateStorageClass=Auto  FilterContinuousStateAttributes=''  FilterStateMustResolveToSignalObject=off  FilterRTWStateStorageClass=Auto  DifferentiatorICPrevScaledInput=0  DifferentiatorOutMin=[]  DifferentiatorOutMax=[]
  Discrete PID Controller1 : simulink/Continuous/PID Controller  Controller=P  TimeDomain=Discrete-time  SampleTime=Ts  IntegratorMethod=Forward Euler  FilterMethod=Forward Euler  Form=Parallel  UseFilter=on  ControllerParametersSource=internal  P=RollPitchKp  I=0.0227534008426031  D=RollPitchKd  N=50  InitialConditionSource=internal  InitialConditionForIntegrator=0  InitialConditionForFilter=0  ExternalReset=none  LimitOutput=on  UpperSaturationLimit=RollPitchRateMax  LowerSaturationLimit=-RollPitchRateMax  LinearizeAsGain=off  AntiWindupMode=clamping  Kb=1  TrackingMode=off  Kt=1  PParamMin=[]  PParamMax=[]  IParamMin=[]  IParamMax=[]  DParamMin=[]  DParamMax=[]  NParamMin=[]  NParamMax=[]  KbParamMin=[]  KbParamMax=[]  KtParamMin=[]  KtParamMax=[]  POutMin=[]  POutMax=[]  IOutMin=[]  IOutMax=[]  DOutMin=[]  DOutMax=[]  NOutMin=[]  NOutMax=[]  KbOutMin=[]  KbOutMax=[]  KtOutMin=[]  KtOutMax=[]  IntegratorOutMin=[]  IntegratorOutMax=[]  FilterOutMin=[]  FilterOutMax=[]  SumOutMin=[]  SumOutMax=[]  SumI1OutMin=[]  SumI1OutMax=[]  SumI2OutMin=[]  SumI2OutMax=[]  SumI3OutMin=[]  SumI3OutMax=[]  SumDOutMin=[]  SumDOutMax=[]  SaturationOutMin=[]  SaturationOutMax=[]  IntegratorContinuousStateAttributes=''  IntegratorStateMustResolveToSignalObject=off  IntegratorRTWStateStorageClass=Auto  FilterContinuousStateAttributes=''  FilterStateMustResolveToSignalObject=off  FilterRTWStateStorageClass=Auto  DifferentiatorICPrevScaledInput=0  DifferentiatorOutMin=[]  DifferentiatorOutMax=[]
  Scale roll2 : Gain  Gain=RollPitchMax
  Selector : Selector  InputPortWidth=3  IndexOptions=Index vector (dialog)  Indices=[1]  OutputSizes=1
  Selector3 : Selector  InputPortWidth=3  IndexOptions=Index vector (dialog)  Indices=[1]  OutputSizes=1
  Sum : Sum  Inputs=|+-
  Sum3 : Sum  Inputs=|+-
  RollPWM : Outport
  wires:
  BUS/1 -> Bus Selector1/1
  Bus Selector1/2 -> Selector/1  "<dRPY>"
  Selector/1 -> Sum/2  "dRoll"
  Discrete PID Controller/1 -> RollPWM/1  "AttRollY"
  RollRef/1 -> Scale roll2/1
  Sum/1 -> Discrete PID Controller/1
  Bus Selector1/1 -> Selector3/1  "<RPY>"
  Discrete PID Controller1/1 -> Sum/1  "AttRollRateRef"
  Selector3/1 -> Sum3/2
  Sum3/1 -> Discrete PID Controller1/1
  Scale roll2/1 -> Sum3/1  "AttRollRef"

== system ModelRikiRollCalib/Ctrl/RollPitchCtrl/Yaw Controller ==
  BUS : Inport
  YawRef : Inport  Port=2
  Bus Selector1 : BusSelector  OutputSignals=dRPY
  Discrete PID Controller : simulink/Continuous/PID Controller  Controller=PI  TimeDomain=Discrete-time  SampleTime=Ts  IntegratorMethod=Forward Euler  FilterMethod=Forward Euler  Form=Parallel  UseFilter=on  ControllerParametersSource=internal  P=YawRateKp  I=YawRateKi  D=0  N=10  InitialConditionSource=internal  InitialConditionForIntegrator=0  InitialConditionForFilter=0  ExternalReset=none  LimitOutput=on  UpperSaturationLimit=0.2  LowerSaturationLimit=-0.2  LinearizeAsGain=off  AntiWindupMode=clamping  Kb=1  TrackingMode=off  Kt=1  PParamMin=[]  PParamMax=[]  IParamMin=[]  IParamMax=[]  DParamMin=[]  DParamMax=[]  NParamMin=[]  NParamMax=[]  KbParamMin=[]  KbParamMax=[]  KtParamMin=[]  KtParamMax=[]  POutMin=[]  POutMax=[]  IOutMin=[]  IOutMax=[]  DOutMin=[]  DOutMax=[]  NOutMin=[]  NOutMax=[]  KbOutMin=[]  KbOutMax=[]  KtOutMin=[]  KtOutMax=[]  IntegratorOutMin=[]  IntegratorOutMax=[]  FilterOutMin=[]  FilterOutMax=[]  SumOutMin=[]  SumOutMax=[]  SumI1OutMin=[]  SumI1OutMax=[]  SumI2OutMin=[]  SumI2OutMax=[]  SumI3OutMin=[]  SumI3OutMax=[]  SumDOutMin=[]  SumDOutMax=[]  SaturationOutMin=[]  SaturationOutMax=[]  IntegratorContinuousStateAttributes=''  IntegratorStateMustResolveToSignalObject=off  IntegratorRTWStateStorageClass=Auto  FilterContinuousStateAttributes=''  FilterStateMustResolveToSignalObject=off  FilterRTWStateStorageClass=Auto  DifferentiatorICPrevScaledInput=0  DifferentiatorOutMin=[]  DifferentiatorOutMax=[]
  Scale roll2 : Gain  Gain=YawRateMax
  Selector : Selector  InputPortWidth=3  IndexOptions=Index vector (dialog)  Indices=[3]  OutputSizes=1
  Sum : Sum  Inputs=|+-
  YawPWM : Outport
  wires:
  Scale roll2/1 -> Sum/1
  Sum/1 -> Discrete PID Controller/1
  YawRef/1 -> Scale roll2/1
  Discrete PID Controller/1 -> YawPWM/1  "YawInput"
  Selector/1 -> Sum/2  "dYaw"
  Bus Selector1/1 -> Selector/1  "<dRPY>"
  BUS/1 -> Bus Selector1/1

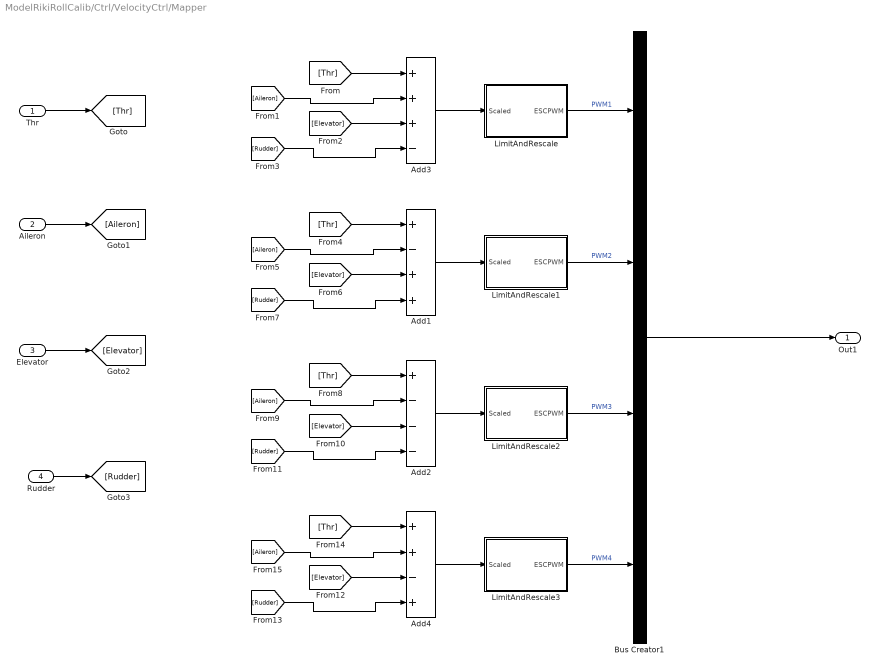
== system ModelRikiRollCalib/Ctrl/VelocityCtrl/Mapper ==
  Thr : Inport
  Aileron : Inport  Port=2
  Elevator : Inport  Port=3
  Rudder : Inport  Port=4
  Add1 : Sum  Inputs=+-++
  Add2 : Sum  Inputs=+---
  Add3 : Sum  Inputs=+++-
  Add4 : Sum  Inputs=++-+
  Bus Creator1 : BusCreator  Inputs=4
  LimitAndRescale : Subsystem
  LimitAndRescale1 : Subsystem
  LimitAndRescale2 : Subsystem
  LimitAndRescale3 : Subsystem
  Out1 : Outport
  wires:
  LimitAndRescale3/1(ESCPWM) -> Bus Creator1/4  "PWM4"
  Add4/1 -> LimitAndRescale3/1(Scaled)
  LimitAndRescale2/1(ESCPWM) -> Bus Creator1/3  "PWM3"
  Add2/1 -> LimitAndRescale2/1(Scaled)
  Bus Creator1/1 -> Out1/1
  LimitAndRescale/1(ESCPWM) -> Bus Creator1/1  "PWM1"
  Add3/1 -> LimitAndRescale/1(Scaled)
  LimitAndRescale1/1(ESCPWM) -> Bus Creator1/2  "PWM2"
  Thr/1 -> [Thr]
  Aileron/1 -> [Aileron]
  Elevator/1 -> [Elevator]
  Rudder/1 -> [Rudder]
  [Thr] -> Add3/1
  [Aileron] -> Add3/2
  [Elevator] -> Add3/3
  [Rudder] -> Add3/4
  Add1/1 -> LimitAndRescale1/1(Scaled)
  [Thr] -> Add1/1
  [Aileron] -> Add1/2
  [Elevator] -> Add1/3
  [Rudder] -> Add1/4
  [Thr] -> Add2/1
  [Aileron] -> Add2/2
  [Elevator] -> Add2/3
  [Rudder] -> Add2/4
  [Thr] -> Add4/1
  [Aileron] -> Add4/2
  [Elevator] -> Add4/3
  [Rudder] -> Add4/4

== system ModelRikiRollCalib/Ctrl/VelocityCtrl/Pitch Controller ==
  BUS : Inport
  PitchRef : Inport  Port=2
  Bus Selector2 : BusSelector  OutputSignals=RPY,dRPY
  Discrete PID Controller : simulink/Continuous/PID Controller  Controller=PI  TimeDomain=Discrete-time  SampleTime=Ts  IntegratorMethod=Forward Euler  FilterMethod=Forward Euler  Form=Parallel  UseFilter=on  ControllerParametersSource=internal  P=RollPitchRateKp  I=RollPitchRateKi  D=0  N=50  InitialConditionSource=internal  InitialConditionForIntegrator=0  InitialConditionForFilter=0  ExternalReset=none  LimitOutput=on  UpperSaturationLimit=0.2  LowerSaturationLimit=-0.2  LinearizeAsGain=off  AntiWindupMode=clamping  Kb=1  TrackingMode=off  Kt=1  PParamMin=[]  PParamMax=[]  IParamMin=[]  IParamMax=[]  DParamMin=[]  DParamMax=[]  NParamMin=[]  NParamMax=[]  KbParamMin=[]  KbParamMax=[]  KtParamMin=[]  KtParamMax=[]  POutMin=[]  POutMax=[]  IOutMin=[]  IOutMax=[]  DOutMin=[]  DOutMax=[]  NOutMin=[]  NOutMax=[]  KbOutMin=[]  KbOutMax=[]  KtOutMin=[]  KtOutMax=[]  IntegratorOutMin=[]  IntegratorOutMax=[]  FilterOutMin=[]  FilterOutMax=[]  SumOutMin=[]  SumOutMax=[]  SumI1OutMin=[]  SumI1OutMax=[]  SumI2OutMin=[]  SumI2OutMax=[]  SumI3OutMin=[]  SumI3OutMax=[]  SumDOutMin=[]  SumDOutMax=[]  SaturationOutMin=[]  SaturationOutMax=[]  IntegratorContinuousStateAttributes=''  IntegratorStateMustResolveToSignalObject=off  IntegratorRTWStateStorageClass=Auto  FilterContinuousStateAttributes=''  FilterStateMustResolveToSignalObject=off  FilterRTWStateStorageClass=Auto  DifferentiatorICPrevScaledInput=0  DifferentiatorOutMin=[]  DifferentiatorOutMax=[]
  Discrete PID Controller1 : simulink/Continuous/PID Controller  Controller=P  TimeDomain=Discrete-time  SampleTime=Ts  IntegratorMethod=Forward Euler  FilterMethod=Forward Euler  Form=Parallel  UseFilter=on  ControllerParametersSource=internal  P=RollPitchKp  I=0.0227534008426031  D=0  N=50  InitialConditionSource=internal  InitialConditionForIntegrator=0  InitialConditionForFilter=0  ExternalReset=none  LimitOutput=on  UpperSaturationLimit=RollPitchRateMax  LowerSaturationLimit=-RollPitchRateMax  LinearizeAsGain=off  AntiWindupMode=clamping  Kb=1  TrackingMode=off  Kt=1  PParamMin=[]  PParamMax=[]  IParamMin=[]  IParamMax=[]  DParamMin=[]  DParamMax=[]  NParamMin=[]  NParamMax=[]  KbParamMin=[]  KbParamMax=[]  KtParamMin=[]  KtParamMax=[]  POutMin=[]  POutMax=[]  IOutMin=[]  IOutMax=[]  DOutMin=[]  DOutMax=[]  NOutMin=[]  NOutMax=[]  KbOutMin=[]  KbOutMax=[]  KtOutMin=[]  KtOutMax=[]  IntegratorOutMin=[]  IntegratorOutMax=[]  FilterOutMin=[]  FilterOutMax=[]  SumOutMin=[]  SumOutMax=[]  SumI1OutMin=[]  SumI1OutMax=[]  SumI2OutMin=[]  SumI2OutMax=[]  SumI3OutMin=[]  SumI3OutMax=[]  SumDOutMin=[]  SumDOutMax=[]  SaturationOutMin=[]  SaturationOutMax=[]  IntegratorContinuousStateAttributes=''  IntegratorStateMustResolveToSignalObject=off  IntegratorRTWStateStorageClass=Auto  FilterContinuousStateAttributes=''  FilterStateMustResolveToSignalObject=off  FilterRTWStateStorageClass=Auto  DifferentiatorICPrevScaledInput=0  DifferentiatorOutMin=[]  DifferentiatorOutMax=[]
  Scale roll1 : Gain  Gain=RollPitchMax
  Selector1 : Selector  InputPortWidth=3  IndexOptions=Index vector (dialog)  Indices=[2]  OutputSizes=1
  Selector2 : Selector  InputPortWidth=3  IndexOptions=Index vector (dialog)  Indices=[2]  OutputSizes=1
  Sum1 : Sum  Inputs=|+-
  Sum3 : Sum  Inputs=|+-
  PitchPWM : Outport
  wires:
  Scale roll1/1 -> Sum3/1
  Sum3/1 -> Discrete PID Controller1/1
  Selector1/1 -> Sum3/2
  Discrete PID Controller1/1 -> Sum1/1
  Bus Selector2/1 -> Selector1/1  "<RPY>"
  Sum1/1 -> Discrete PID Controller/1
  PitchRef/1 -> Scale roll1/1
  Discrete PID Controller/1 -> PitchPWM/1
  Selector2/1 -> Sum1/2  "dRoll"
  Bus Selector2/2 -> Selector2/1  "<dRPY>"
  BUS/1 -> Bus Selector2/1

== system ModelRikiRollCalib/Ctrl/VelocityCtrl/Roll Controller ==
  BUS : Inport
  RollRef : Inport  Port=2
  Bus Selector1 : BusSelector  OutputSignals=RPY,dRPY
  Discrete PID Controller : simulink/Continuous/PID Controller  Controller=PI  TimeDomain=Discrete-time  SampleTime=Ts  IntegratorMethod=Forward Euler  FilterMethod=Forward Euler  Form=Parallel  UseFilter=on  ControllerParametersSource=internal  P=RollPitchRateKp  I=RollPitchRateKi  D=0  N=50  InitialConditionSource=internal  InitialConditionForIntegrator=0  InitialConditionForFilter=0  ExternalReset=none  LimitOutput=on  UpperSaturationLimit=0.2  LowerSaturationLimit=-0.2  LinearizeAsGain=off  AntiWindupMode=clamping  Kb=1  TrackingMode=off  Kt=1  PParamMin=[]  PParamMax=[]  IParamMin=[]  IParamMax=[]  DParamMin=[]  DParamMax=[]  NParamMin=[]  NParamMax=[]  KbParamMin=[]  KbParamMax=[]  KtParamMin=[]  KtParamMax=[]  POutMin=[]  POutMax=[]  IOutMin=[]  IOutMax=[]  DOutMin=[]  DOutMax=[]  NOutMin=[]  NOutMax=[]  KbOutMin=[]  KbOutMax=[]  KtOutMin=[]  KtOutMax=[]  IntegratorOutMin=[]  IntegratorOutMax=[]  FilterOutMin=[]  FilterOutMax=[]  SumOutMin=[]  SumOutMax=[]  SumI1OutMin=[]  SumI1OutMax=[]  SumI2OutMin=[]  SumI2OutMax=[]  SumI3OutMin=[]  SumI3OutMax=[]  SumDOutMin=[]  SumDOutMax=[]  SaturationOutMin=[]  SaturationOutMax=[]  IntegratorContinuousStateAttributes=''  IntegratorStateMustResolveToSignalObject=off  IntegratorRTWStateStorageClass=Auto  FilterContinuousStateAttributes=''  FilterStateMustResolveToSignalObject=off  FilterRTWStateStorageClass=Auto  DifferentiatorICPrevScaledInput=0  DifferentiatorOutMin=[]  DifferentiatorOutMax=[]
  Discrete PID Controller1 : simulink/Continuous/PID Controller  Controller=P  TimeDomain=Discrete-time  SampleTime=Ts  IntegratorMethod=Forward Euler  FilterMethod=Forward Euler  Form=Parallel  UseFilter=on  ControllerParametersSource=internal  P=RollPitchKp  I=0.0227534008426031  D=0  N=50  InitialConditionSource=internal  InitialConditionForIntegrator=0  InitialConditionForFilter=0  ExternalReset=none  LimitOutput=on  UpperSaturationLimit=RollPitchRateMax  LowerSaturationLimit=-RollPitchRateMax  LinearizeAsGain=off  AntiWindupMode=clamping  Kb=1  TrackingMode=off  Kt=1  PParamMin=[]  PParamMax=[]  IParamMin=[]  IParamMax=[]  DParamMin=[]  DParamMax=[]  NParamMin=[]  NParamMax=[]  KbParamMin=[]  KbParamMax=[]  KtParamMin=[]  KtParamMax=[]  POutMin=[]  POutMax=[]  IOutMin=[]  IOutMax=[]  DOutMin=[]  DOutMax=[]  NOutMin=[]  NOutMax=[]  KbOutMin=[]  KbOutMax=[]  KtOutMin=[]  KtOutMax=[]  IntegratorOutMin=[]  IntegratorOutMax=[]  FilterOutMin=[]  FilterOutMax=[]  SumOutMin=[]  SumOutMax=[]  SumI1OutMin=[]  SumI1OutMax=[]  SumI2OutMin=[]  SumI2OutMax=[]  SumI3OutMin=[]  SumI3OutMax=[]  SumDOutMin=[]  SumDOutMax=[]  SaturationOutMin=[]  SaturationOutMax=[]  IntegratorContinuousStateAttributes=''  IntegratorStateMustResolveToSignalObject=off  IntegratorRTWStateStorageClass=Auto  FilterContinuousStateAttributes=''  FilterStateMustResolveToSignalObject=off  FilterRTWStateStorageClass=Auto  DifferentiatorICPrevScaledInput=0  DifferentiatorOutMin=[]  DifferentiatorOutMax=[]
  Scale roll2 : Gain  Gain=RollPitchMax
  Selector : Selector  InputPortWidth=3  IndexOptions=Index vector (dialog)  Indices=[1]  OutputSizes=1
  Selector3 : Selector  InputPortWidth=3  IndexOptions=Index vector (dialog)  Indices=[1]  OutputSizes=1
  Sum : Sum  Inputs=|+-
  Sum3 : Sum  Inputs=|+-
  RollPWM : Outport
  wires:
  Scale roll2/1 -> Sum3/1
  Sum3/1 -> Discrete PID Controller1/1
  Selector3/1 -> Sum3/2
  Discrete PID Controller1/1 -> Sum/1
  Bus Selector1/1 -> Selector3/1  "<RPY>"
  Sum/1 -> Discrete PID Controller/1
  RollRef/1 -> Scale roll2/1
  Discrete PID Controller/1 -> RollPWM/1
  Selector/1 -> Sum/2  "dRoll"
  Bus Selector1/2 -> Selector/1  "<dRPY>"
  BUS/1 -> Bus Selector1/1

== system ModelRikiRollCalib/Ctrl/VelocityCtrl/Subsystem ==
  VertVellRef : Inport
  VertVel : Inport  Port=2
  Bias : Bias  Bias=-0.5
  Bias1 : Bias  Bias=AltRateBias
  Dead Zone : DeadZone  LowerValue=-0.1  UpperValue=0.1  SaturateOnIntegerOverflow=on
  Discrete PID Controller1 : simulink/Continuous/PID Controller  Controller=PI  TimeDomain=Discrete-time  SampleTime=Ts  IntegratorMethod=Forward Euler  FilterMethod=Forward Euler  Form=Parallel  UseFilter=on  ControllerParametersSource=internal  P=AltRateKp  I=AltRateKi  D=0  N=50  InitialConditionSource=internal  InitialConditionForIntegrator=0  InitialConditionForFilter=0  ExternalReset=none  LimitOutput=on  UpperSaturationLimit=0.5  LowerSaturationLimit=-0.5  LinearizeAsGain=off  AntiWindupMode=clamping  Kb=1  TrackingMode=off  Kt=1  PParamMin=[]  PParamMax=[]  IParamMin=[]  IParamMax=[]  DParamMin=[]  DParamMax=[]  NParamMin=[]  NParamMax=[]  KbParamMin=[]  KbParamMax=[]  KtParamMin=[]  KtParamMax=[]  POutMin=[]  POutMax=[]  IOutMin=[]  IOutMax=[]  DOutMin=[]  DOutMax=[]  NOutMin=[]  NOutMax=[]  KbOutMin=[]  KbOutMax=[]  KtOutMin=[]  KtOutMax=[]  IntegratorOutMin=[]  IntegratorOutMax=[]  FilterOutMin=[]  FilterOutMax=[]  SumOutMin=[]  SumOutMax=[]  SumI1OutMin=[]  SumI1OutMax=[]  SumI2OutMin=[]  SumI2OutMax=[]  SumI3OutMin=[]  SumI3OutMax=[]  SumDOutMin=[]  SumDOutMax=[]  SaturationOutMin=[]  SaturationOutMax=[]  IntegratorContinuousStateAttributes=''  IntegratorStateMustResolveToSignalObject=off  IntegratorRTWStateStorageClass=Auto  FilterContinuousStateAttributes=''  FilterStateMustResolveToSignalObject=off  FilterRTWStateStorageClass=Auto  DifferentiatorICPrevScaledInput=0  DifferentiatorOutMin=[]  DifferentiatorOutMax=[]
  Scale Vel : Gain  Gain=AltRateMax*2
  Sum3 : Sum  Inputs=|+-
  Out1 : Outport
  wires:
  VertVellRef/1 -> Bias/1
  Bias1/1 -> Out1/1
  Scale Vel/1 -> Sum3/1
  VertVel/1 -> Sum3/2
  Discrete PID Controller1/1 -> Bias1/1
  Sum3/1 -> Discrete PID Controller1/1
  Bias/1 -> Dead Zone/1
  Dead Zone/1 -> Scale Vel/1
